simulink library "Input_Air"  (R2018b)
settings: Solver=ode45  StartTime=0.0  StopTime=10.0  RelTol=1e-3  EnableMultiTasking=on
settings Model: Creator=lena.frank  LastModifiedBy=P41573
settings DataIOCC: LimitDataPoints=on  SaveFormat=Array  SignalLoggingSaveFormat=ModelDataLogs
settings OptimizationCC: ExpressionDepthLimit=2147483647  LifeSpan=inf
settings DebuggingCC: UnderspecifiedInitializationDetection=Classic  MergeDetectMultiDrivingBlocksExec=none  SolverPrmCheckMsg=warning  FcnCallInpInsideContextMsg=warning  StateNameClashWarn=warning  SFUnexpectedBacktrackingDiag=warning  SFNoUnconditionalDefaultTransitionDiag=warning  SFExecutionAtInitializationDiag=none
settings HardwareCC: ProdBitPerPointer=32  ProdBitPerSizeT=32  ProdBitPerPtrDiffT=32  ProdLargestAtomicFloat=None  ProdIntDivRoundTo=Undefined  ProdEndianess=Unspecified  ProdWordSize=32  ProdHWDeviceType=32-bit Generic
settings ModelReferenceCC: PropagateSignalLabelsOutOfModel=off
settings SFSimCC: SimUseLocalCustomCode=off
settings RTWCC: RTWUseLocalCustomCode=off
settings CodeAppCC: StateflowObjectComments=on
settings GRTTargetCC: TargetLangStandard=C89/C90 (ANSI)  GeneratePreprocessorConditionals=Disable all  CombineOutputUpdateFcns=off  GRTInterface=on
settings ConfigComp: CovMetricSettings=dw  CovHtmlReporting=on  CovSaveCumulativeToWorkspaceVar=on  CovSaveSingleToWorkspaceVar=on  CovExternalEMLEnable=off

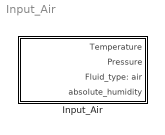
== system Input_Air ==
  Input_Air : Subsystem  mask(Input_Air){T=20, p=1e5, x=0.005}
      mask prompts: T "temperature (scalar or vector) [°C]"; p "pressure [Pa]"; x "absolute humidity of moist air [kg water/kg dry air]"
      mask help:
      | Input block for the material "Air"
      |
      | The relevant inputs for the calculation of the block can be specified as parameter in the mask
      mask Help: web(fullfile(path_carnot('help'),'input_material.html'),'-helpbrowser')

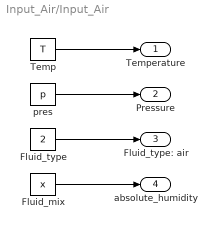
== system Input_Air/Input_Air ==
  Fluid_mix : Constant  Value=x
  Fluid_type : Constant  Value=2
  Temp : Constant  Value=T
  pres : Constant  Value=p
  Temperature : Outport
  Pressure : Outport  Port=2
  Fluid_type: air : Outport  Port=3
  absolute_humidity : Outport  Port=4
  wires:
  pres/1 -> Pressure/1
  Temp/1 -> Temperature/1
  Fluid_type/1 -> Fluid_type: air/1
  Fluid_mix/1 -> absolute_humidity/1
